simulink model "dcmtr_SimVsTest"  (R2021b)
settings: Solver=VariableStepAuto  StartTime=0.0  StopTime=10.0  RelTol=1e-3
undefined symbols (not defined in the file): DCMtr_b, DCMtr_Fs, DCMtr_J, DCMtr_K, DCMtr_L, DCMtr_R
libraries: fl_lib x6, nesl_utility x3, simulink_extras x2, ee_lib x1
CloseFcn:
  | clear
settings Model: Creator=smuckati  LastModifiedBy=smuckati
settings DebuggingCC: ParameterPrecisionLossMsg=none

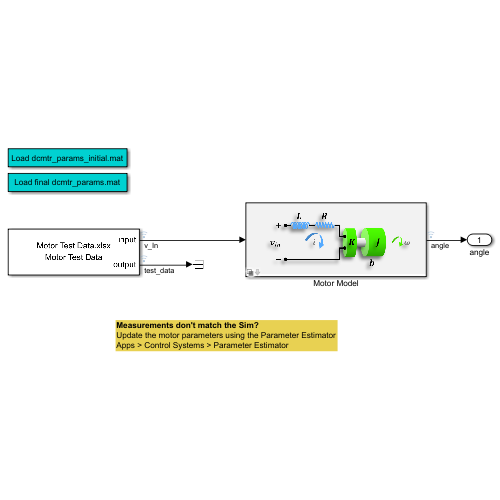
[thumbnail: Simulink's stored preview of the top-level diagram]
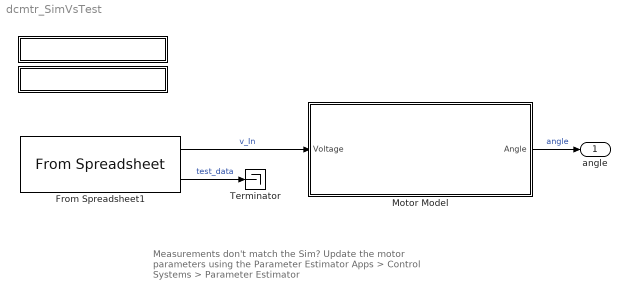
== system dcmtr_SimVsTest ==
  note: Measurements don't match the Sim?
      | Update the motor parameters using the Parameter Estimator
      | Apps > Control Systems > Parameter Estimator
  " " : Subsystem
      settings: OpenFcn=|
      | clear
      | try
      | load('dcmtr_params_initial.mat');
      | msgbox('Variables loaded to MATLAB workspace')
      | catch
      | error('Error loading parameters')
      | end
      mask Display: disp('Load dcmtr_params_initial.mat')
  "  " : Subsystem
      settings: OpenFcn=|
      | clear
      | try
      |     load('dcmtr_params.mat');
      |     msgbox('Variables loaded to MATLAB workspace')
      | catch
      |     error('Error loading parameters')
      | end
      mask Display: disp('Load final dcmtr_params.mat')
  From Spreadsheet1 : FromSpreadsheet  FileName=Motor Test Data.xlsx  SheetName=Motor Test Data  Range=A1:C80002
  Motor Model : Subsystem  Variant=on  VariantControlMode=label  LabelModeActiveChoice=Simulink  mask(DC Motor){varChoice=Simulink, K=DCMtr_K, R=DCMtr_R, L=DCMtr_L, b=DCMtr_b, J=DCMtr_J, Fs=DCMtr_Fs}
      mask prompts: varChoice "Select Model Type"; K "Torque Constant"; R "Armature Resistance"; L "Armature Inductance"; b "Damping Coeffecient"; J "Rotor Inertia"; Fs "Friction Torque"
      mask help: This block simulates a basic brushed DC Motor with voltage input and rotor angle in as the output.
      mask init:
      | choice = get_param(gcb,'varChoice');
      | vssBlk = gcb;
      | oldVariant = get_param(gcb,'LabelModeActiveChoice');
      | if strcmp(choice,'Simulink')
      |     
      |     set_param(vssBlk, 'LabelModeActiveChoice', 'Simulink');
      | else
      |     
      |     set_param(vssBlk, 'LabelModeActiveChoice', 'Simscape');
      | end
      mask TypeOptions varChoice: Simulink | Simscape
      mask DialogControl ModelType Prompt: Model Used
      mask Display: image('$imagefile'); % Use "Edit Image" on toolstrip to change.
  Terminator : Terminator
  angle : Outport
  wires:
  From Spreadsheet1/2 -> Terminator/1  "test_data"
  From Spreadsheet1/1 -> Motor Model/1(Voltage)  "v_In"
  Motor Model/1(Angle) -> angle/1  "angle"

== system dcmtr_SimVsTest/  ==

== system dcmtr_SimVsTest/   ==

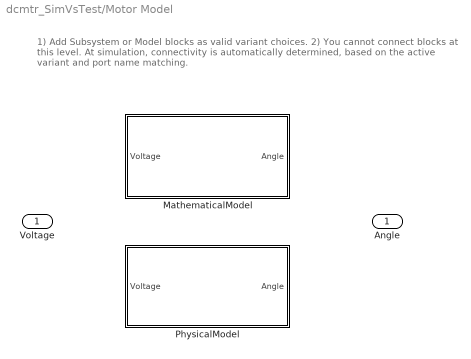
== system dcmtr_SimVsTest/Motor Model ==
  note: 1) Add Subsystem or Model blocks as valid variant choices.
      | 2) You cannot connect blocks at this level. At simulation, connectivity is automatically
      | determined, based on the active variant and port name matching.
  Voltage : Inport
  MathematicalModel : Subsystem  VariantControl=Simulink
  PhysicalModel : Subsystem  VariantControl=Simscape
  Angle : Outport

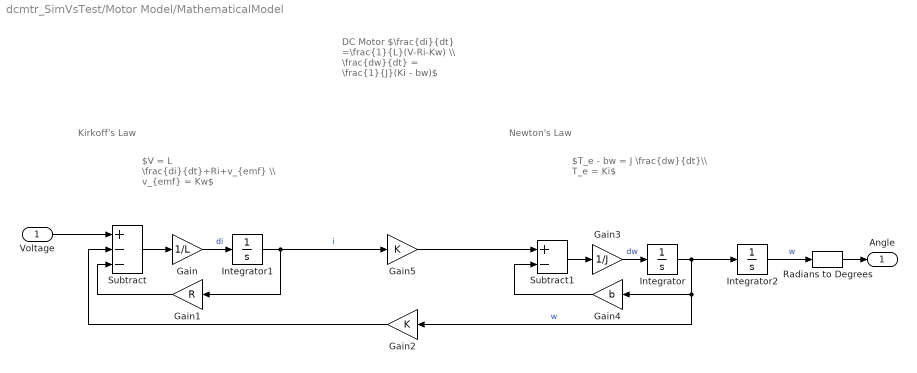
== system dcmtr_SimVsTest/Motor Model/MathematicalModel ==
  note: Newton's Law
  note: $T_e - bw = J \frac{dw}{dt}\\ T_e = Ki$
  note: Kirkoff's Law
  note: $V = L \frac{di}{dt}+Ri+v_{emf} \\ v_{emf} = Kw$
  note: DC Motor
      | $\frac{di}{dt} =\frac{1}{L}(V-Ri-Kw) \\ \frac{dw}{dt} = \frac{1}{J}(Ki - bw)$
  Voltage : Inport
  Gain : Gain  Gain=1/L
  Gain1 : Gain  Gain=R
  Gain2 : Gain  Gain=K
  Gain3 : Gain  Gain=1/J
  Gain4 : Gain  Gain=b
  Gain5 : Gain  Gain=K
  Integrator : Integrator
  Integrator1 : Integrator
  Integrator2 : Integrator
  Radians to Degrees : simulink_extras/Transformations/Radians to Degrees
  Subtract : Sum  Inputs=+--
  Subtract1 : Sum  Inputs=+-
  Angle : Outport  VectorParamsAs1DForOutWhenUnconnected=off
  wires:
  Gain1/1 -> Subtract/3
  Integrator1/1 -> Gain5/1, Gain1/1  "i"
  Integrator/1 -> Integrator2/1, Gain2/1, Gain4/1  "w"
  Gain2/1 -> Subtract/2
  Subtract1/1 -> Gain3/1
  Gain3/1 -> Integrator/1  "dw"
  Gain4/1 -> Subtract1/2
  Gain5/1 -> Subtract1/1
  Subtract/1 -> Gain/1
  Gain/1 -> Integrator1/1  "di"
  Voltage/1 -> Subtract/1
  Integrator2/1 -> Radians to Degrees/1  "w"
  Radians to Degrees/1 -> Angle/1

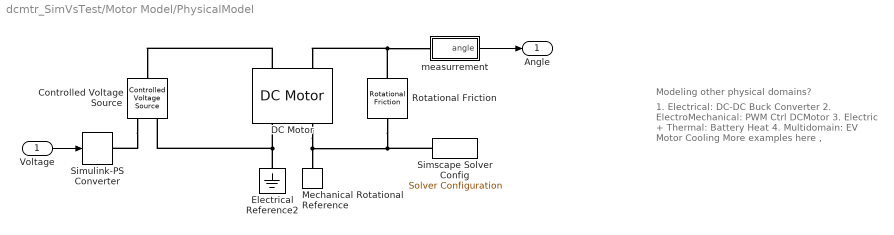
== system dcmtr_SimVsTest/Motor Model/PhysicalModel ==
  note: 1. Electrical: DC-DC Buck Converter
      | 2. ElectroMechanical: PWM Ctrl DCMotor
      | 3. Electric + Thermal: Battery Heat
      | 4. Multidomain: EV Motor Cooling
      |
      | More examples here ,
  note: Modeling other physical domains?
  Voltage : Inport
  Controlled Voltage Source : fl_lib/Electrical/Electrical Sources/Controlled Voltage Source
  DC Motor : ee_lib/Electromechanical/Brushed Motors/DC Motor  field_option=ee.enum.field_option.pm  Rf=100 Ohm  Lf=1 H  Laf=0.15 H  If0=0 A  parameterization=ee.enum.dcparam_option.circuit_param  Ra=R Ohm  La=L H  emf_or_torque=ee.enum.emf_or_torque.ki  Kv=K V/(rad/s)  Ki=K N*m/A  T_stall=57/16 in*lbf  w_max=62.5 rpm  w_rated=1.5e+04 rpm  P_rated=0.08 W  V_rated=5 V  lam_param=ee.enum.lam_param.damping  i_noload=0 A  V_i_noload=1.5 V  J=J kg*m^2  lam=b N*m/(rad/s)  speed0=0 rpm  enable_fault_armature=simscape.enum.onoff.off  rev_faulted=1 / 3  G_faulted_armature=1e-5 S  fault_trigger_armature=ee.enum.faults.faultTrigger.temporal  t_fault_armature=1 s  max_permissible_current_armature=inf A  t_fail_on_current_armature=1 s  enable_fault_field=simscape.enum.onoff.off  G_faulted_field=1e-5 S  fault_trigger_field=ee.enum.faults.faultTrigger.temporal  t_fault_field=1 s  max_permissible_current_field=inf A  t_fail_on_current_field=1 s  fault_action=simscape.enum.assert.action.none  alpha=3.93e-3 1/K  Tmeas=25 degC  thermal_mass=100 J/K  initial_temperature=25 degC
  Electrical Reference2 : fl_lib/Electrical/Electrical Elements/Electrical Reference
  Mechanical Rotational Reference : fl_lib/Mechanical/Rotational Elements/Mechanical Rotational Reference
  Rotational Friction : fl_lib/Mechanical/Rotational Elements/Rotational Friction  brkwy_trq=Fs N*m  brkwy_vel=0.001 rad/s  Col_trq=0.001 N*m  visc_coef=0.001 N*m/(rad/s)  w_specify=off  w_priority=None  w=0 rad/s  w_nominal_specify=off  w_nominal_unit=rad/s  w_nominal_value=1  t_specify=off  t_priority=None  t=0 N*m  t_nominal_specify=off  t_nominal_unit=N*m  t_nominal_value=1
  Simscape Solver Config : nesl_utility/Solver Configuration  PhysicalDomain=network_engine_domain  SubClassName=solver  LeftPortType=input  RightPortType=generic  Tones=[]  Harmonics=[]  SimulateNoise=off  Profile=off  UseLocalSampling=off  EnableSwitchedLinearOptims=on  FrequencyDomain=off  UseCCode=off  RelTol=0.001  AbsTol=1e-06  MinStep=1e-09  ToWorkspace=off  RevertToSquareIcSolve=off  NumHomotopyIterations=100  PhasorMode=off  PhasorModeNumHarmonics=1  DoDC=off  ResidualTolerance=1e-9  UseLocalSolver=off  LocalSolverChoice=NE_BACKWARD_EULER_ADVANCER  LocalSolverSampleTime=0.00125  DoFixedCost=off  MaxNonlinIter=3  MaxModeIter=2  ComputeImpulses=off  ImpulseIterations=2  LinearAlgebra=Sparse  EquationFormulation=NE_TIME_EF  DelaysMemoryBudget=1024  AutomaticFiltering=on  FilteringTimeConstant=0.001  PartitionStorageMethod=AS_NEEDED  PartitionMemoryBudget=1024  PartitionMethod=FAST
  Simulink-PS Converter : nesl_utility/Simulink-PS Converter  PhysicalDomain=network_engine_domain  SubClassName=ps_input  LeftPortType=input  RightPortType=output  PseudoPeriodic=off  Frequencies=[]  NoiseDistribution=none  NoiseParameters=[]  Unit=1  AffineConversion=off  FilteringAndDerivatives=zero  SimscapeFilterOrder=1  InputFilterTimeConstant=.001  UdotUserProvided=0
  measurrement : Subsystem
      mask Display: disp('Sensor')
  Angle : Outport  VectorParamsAs1DForOutWhenUnconnected=off
  wires:
  Voltage/1 -> Simulink-PS Converter/1
  measurrement/1(angle) -> Angle/1
  connections:
  Electrical Reference2/LConn1 -- Controlled Voltage Source/RConn2 -- DC Motor/RConn1
  Controlled Voltage Source/RConn1 -- Simulink-PS Converter/RConn1
  DC Motor/RConn2 -- Mechanical Rotational Reference/LConn1 -- Simscape Solver Config/RConn1 -- Rotational Friction/RConn1
  Rotational Friction/LConn1 -- DC Motor/LConn2 -- measurrement/LConn1
  DC Motor/LConn1 -- Controlled Voltage Source/LConn1

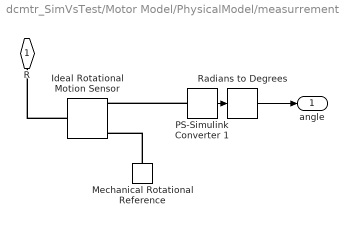
== system dcmtr_SimVsTest/Motor Model/PhysicalModel/measurrement ==
  Ideal Rotational Motion Sensor : fl_lib/Mechanical/Mechanical Sensors/Ideal Rotational Motion Sensor  wrap_angle=simscape.enum.onoff.off  offset=0 rad
  Mechanical Rotational Reference : fl_lib/Mechanical/Rotational Elements/Mechanical Rotational Reference
  PS-Simulink Converter 1 : nesl_utility/PS-Simulink Converter  PhysicalDomain=network_engine_domain  SubClassName=ps_output  LeftPortType=input  RightPortType=output  PseudoPeriodic=off  Frequencies=[]  Unit=rad  AffineConversion=off
  Radians to Degrees : simulink_extras/Transformations/Radians to Degrees
  R : PMIOPort  Side=Left
  angle : Outport
  wires:
  Radians to Degrees/1 -> angle/1
  PS-Simulink Converter 1/1 -> Radians to Degrees/1
  connections:
  Mechanical Rotational Reference/LConn1 -- Ideal Rotational Motion Sensor/RConn1
  Ideal Rotational Motion Sensor/LConn1 -- R/RConn1
  PS-Simulink Converter 1/LConn1 -- Ideal Rotational Motion Sensor/RConn3
